simulink library "alphaZ_ul"  (R2020a)
settings: Solver=VariableStepAuto  StartTime=0.0  StopTime=10.0  RelTol=1e-3
settings Model: Creator=mcobb  LastModifiedBy=John Jr
settings DataIOCC: ReturnWorkspaceOutputs=off
settings DebuggingCC: ArithmeticOperatorsInVariantConditions=warning
settings SFSimCC: CustomCodeUndefinedFunction=UseInterfaceOnly

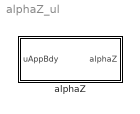
== system alphaZ_ul ==
  alphaZ : Subsystem  TreatAsAtomicUnit=on
      settings: MinAlgLoopOccurrences=on

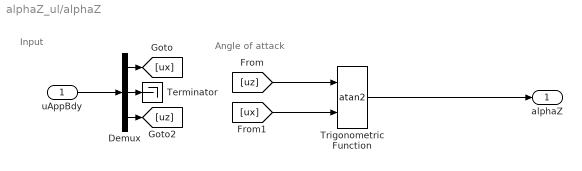
== system alphaZ_ul/alphaZ ==
  note: Angle of attack
  note: Input
  uAppBdy : Inport
  Demux : Demux  Outputs=3
  Terminator : Terminator
  Trigonometric Function : Trigonometry  Operator=atan2
  alphaZ : Outport  VectorParamsAs1DForOutWhenUnconnected=off
  wires:
  uAppBdy/1 -> Demux/1
  Demux/1 -> [ux]
  Demux/2 -> Terminator/1
  Demux/3 -> [uz]
  Trigonometric Function/1 -> alphaZ/1
  [uz] -> Trigonometric Function/1
  [ux] -> Trigonometric Function/2
